simulink model "lissajous"  (R2023b)
settings: Solver=VariableStepAuto  StartTime=0.0  StopTime=10.0  RelTol=1e-3
values from neighbouring files (symbols this model uses):
  a = time_gain * a0    (= 1)    [init.m]
  A = 0.4    [init.m]
  B = 0.4    [init.m]
  b = time_gain * b0    (= 2)    [init.m]
  C = 0.4    [init.m]
  c = time_gain * c0    (= 1.5)    [init.m]
  d = [(21*sin(q6)*(cos(q5)*(cos(q4)*(sin(q1)*sin(q3) - cos(q1)*cos(q2)*cos(q3)) - cos(q1)*sin(q2)*sin(q4)) + sin(q5)*(cos(q3)*sin(q1) + cos(q1)*cos(q2)*sin(q3))))/100 - (21*cos(q6)*(sin(q4)*(sin(q1)*sin(q3) - cos(q1)*cos(q2)*cos(q3)) + cos(q1)*cos(q4)*sin(q2)))/100 - (21*cos(q1)*sin(q2))/50 - (2*sin(q4)*(sin(q1)*sin(q3) - cos(q1)*cos(q2)*cos(q3)))/5 - (2*cos(q1)*cos(q4)*sin(q2))/5 ... (first row only)    [get_position_ee.m]    (also in init.m = 1.57079632679)
  f = pi/3    (= 1.0471975512)    [init.m]
  Lambda_IK = 1*eye(3)    [init.m]
  lev_mar = false    [init.m]
  mu_0 = 1e-1    (= 0.1)    [init.m]
  p0 = [0.4; 0; 0.6]    [init.m]
  q0 = [0.25 ; 0.25; 0.25 ; 0.25; 0.25 ; 0.25; 0.25]    [init.m]
settings Model: Creator=Giorgia  LastModifiedBy=Giorgia

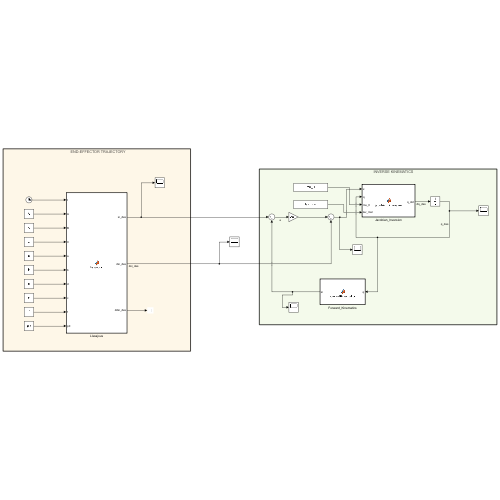
[thumbnail: Simulink's stored preview of the top-level diagram]
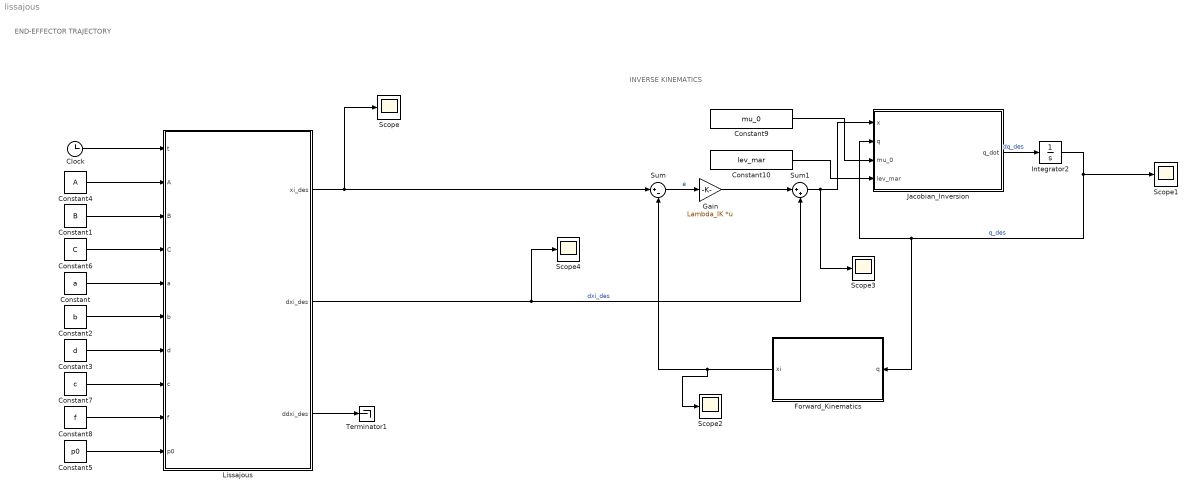
== system lissajous ==
  note: END-EFFECTOR TRAJECTORY
  note: INVERSE KINEMATICS
  Clock : Clock
  Constant : Constant  Value=a
  Constant1 : Constant  Value=B
  Constant10 : Constant  Value=lev_mar
  Constant2 : Constant  Value=b
  Constant3 : Constant  Value=d
  Constant4 : Constant  Value=A
  Constant5 : Constant  Value=p0
  Constant6 : Constant  Value=C
  Constant7 : Constant  Value=c
  Constant8 : Constant  Value=f
  Constant9 : Constant  Value=mu_0
  Forward_Kinematics : MATLAB Function  TreatAsAtomicUnit=on
  Gain : Gain  Gain=Lambda_IK  Multiplication=Matrix(K*u)
  Integrator2 : Integrator  InitialCondition=q0
  Jacobian_Inversion : MATLAB Function  TreatAsAtomicUnit=on
  Lissajous : MATLAB Function  TreatAsAtomicUnit=on
  Scope{,1..4} (5 alike) : Scope
  Sum : Sum  Inputs=|+-
  Sum1 : Sum  Inputs=|++
  Terminator1 : Terminator
  wires:
  Constant/1 -> Lissajous/5(a)
  Constant5/1 -> Lissajous/10(p0)
  Lissajous/3(ddxi_des) -> Terminator1/1
  Clock/1 -> Lissajous/1(t)
  Constant3/1 -> Lissajous/7(d)
  Constant2/1 -> Lissajous/6(b)
  Constant4/1 -> Lissajous/2(A)
  Constant1/1 -> Lissajous/3(B)
  Constant6/1 -> Lissajous/4(C)
  Constant7/1 -> Lissajous/8(c)
  Constant8/1 -> Lissajous/9(f)
  Sum/1 -> Gain/1  "e"
  Lissajous/2(dxi_des) -> Scope4/1, Sum1/2  "dxi_des"
  Sum1/1 -> Scope3/1, Jacobian_Inversion/1(x)
  Constant9/1 -> Jacobian_Inversion/3(mu_0)
  Gain/1 -> Sum1/1
  Jacobian_Inversion/1(q_dot) -> Integrator2/1  "dq_des"
  Constant10/1 -> Jacobian_Inversion/4(lev_mar)
  Forward_Kinematics/1(xi) -> Sum/2, Scope2/1
  Integrator2/1 -> Jacobian_Inversion/2(q), Forward_Kinematics/1(q), Scope1/1  "q_des"
  Lissajous/1(xi_des) -> Sum/1, Scope/1

== matlab function lissajous/Forward_Kinematics ==
  data: q input; xi output
function xi = forwardKinematics(q)
    % q1 = q(1);
    % q2 = q(2);
    % q3 = q(3);
    % q4 = q(4);
    % q5 = q(5);
    % q6 = q(6);
    % q7 = q(7);
    % 
    % T01r = [cos(q1), -sin(q1), 0;
    %        sin(q1) , cos(q1), 0;
    %         0, 0, 1] * [1, 0, 0;
    %                     0, 0, -1;
    %                     0, 1, 0];
    % T01t = [0 0 0.36]';
    % 
    % T12r = [cos(q2), -sin(q2), 0;
    %        sin(q2) , cos(q2), 0;
    %         0, 0, 1] * [1, 0, 0;
    %                     0, 0, 1;
    %                     0, -1, 0];
    % 
    % T23r = [cos(q3), -sin(q3), 0;
    %        sin(q3) , cos(q3), 0;
    %         0, 0, 1] * [1, 0, 0;
    %                     0, 0, 1;
    %                     0, -1, 0]; 
    % 
    % T23t = [0 0 0.42]';
    % 
    % T34r = [cos(q4), -sin(q4), 0;
    %        sin(q4) , cos(q4), 0;
    %         0, 0, 1] * [1, 0, 0;
    %                     0, 0, -1;
    %                     0, 1, 0]; 
    % 
    % T45r = [cos(q5), -sin(q5), 0;
    %        sin(q5) , cos(q5), 0;
    %         0, 0, 1] * [1, 0, 0;
    %                     0, 0, -1;
    %                     0, 1, 0]; 
    % 
    % T45t = [0 0 0.4]';
    % 
    % T56r = [cos(q6), -sin(q6), 0;
    %        sin(q6) , cos(q6), 0;
    %         0, 0, 1] * [1, 0, 0;
    %                     0, 0, 1;
    %                     0, -1, 0];
    % 
    % T67r = [cos(q7), -sin(q7), 0;
    %        sin(q7) , cos(q7), 0;
    %         0, 0, 1];
    % 
    % T67t = [0 0 0.21]';
    % 
    % O33 = zeros(1,3);
    % 
    % T = [T01r, T01t;
    % O33, 1]*[T12r, O33';
    % O33, 1]*[T23r, T23t;
    % O33, 1]*[T34r, O33';
    % O33, 1]*[T45r, T45t;
    % O33,1]*[T56r,  O33';
    % O33, 1]*[T67r, T67t;
    % O33, 1];
    % 
    % 
    % xi = T(1:3,4);

    xi = get_position_ee(q);

== matlab function lissajous/Jacobian_Inversion ==
  settings: updateMethod=DISCRETE
  data: x input; q_dot output size=7; q input; mu_0 input; lev_mar input
function q_dot = jacobian_inversion(x, q, mu_0, lev_mar)
    
    % Getting jacobian and forward kinematics for current guess
    % coder. extrinsic(' get_analytic_jacobian ');
    J = get_analytic_jacobian(q);
    
    % Jacobian inversion
    % J_star = zeros(size(J.')); % preallocating
    % if lev_mar
        % J_star = inv(J.'*J + mu_0*diag(diag(J.'*J)))*J.';
    % else
        % J_star = inv(J(1:3,:));
    % end
    J_star = pinv(J)
    
q_dot = J_star * x;

== matlab function lissajous/Lissajous ==
  data: t input; xi_des output; A input; B input; C input; a input; b input; d input; c input; f input; dxi_des output; ddxi_des output; p0 input
function [xi_des, dxi_des, ddxi_des] = lissajous(t,A,B,C,a,b,d,c,f,p0)
% 
% xi_des = [A*sin(t); B*sin(b*t+d); C*sin(c*t+f)] + p0;
% dxi_des = [A*cos(t); B*b*cos(b*t+d); C*c*cos(c*t+f)];
% ddxi_des = [-A*sin(t); -B*b^2*sin(b*t+d); -C*c^2*sin(c*t+f)];
% 
% xi_des = [0; B*sin(b*t); C*sin(c*t+f)] + p0;
% dxi_des = [0; B*b*cos(b*t); C*c*cos(c*t+f)];
% ddxi_des = [0; -B*b^2*sin(b*t); -C*c^2*sin(c*t+f)];

xi_des = [0; 0.1*cos(t); 0.1*sin(t)] + p0;
dxi_des = [0; -0.1*sin(t); 0.1*cos(t)];
ddxi_des = [0; -0.1*cos(t); -0.1*sin(t)];
